simulink model "hf_point_mass_subsonic_airplane"  (R2024b)
settings: Solver=ode45  StartTime=0.0  StopTime=5*60  RelTol=1e-3  AbsTol=1e-6
values from neighbouring files (symbols this model uses):
  FPS2MPH = 3600/5280    (= 0.681818181818)    [luckep2.m]
  RAD2DEG = 180/pi    (= 57.2957795131)    [luckep2.m]
undefined symbols (not defined in the file or in its folder): gd, ic, params
libraries: simulink_extras x5, dspstat3 x1, simulink x1
(part 2 of 2)

== matlab function hf_point_mass_subsonic_airplane/Vehicle Dynamics/Heading Rate Equation/F_app2/rni/get r_ni ==
  data: bank input; rni output; fpa input; heading input; we input; latitude input; longitude input
function rni = getrni(bank,fpa,heading, we, latitude, longitude)
x = [bank, fpa, heading];
C = [cosd(fpa)*cosd(heading) cosd(fpa)*sind(heading) -sind(fpa)
    sind(bank)*sind(fpa)*cosd(heading) - cosd(bank)*sind(heading) sind(bank)*sind(fpa)*sind(heading) + cosd(bank)*cosd(heading) sind(bank)*cosd(fpa)
    cosd(bank)*sind(fpa)*cosd(heading) + sind(bank)*sind(heading) cosd(bank)*sind(fpa)*sind(heading) - sind(bank)*cosd(heading) cosd(bank)*cosd(fpa)];

mat = C*[(we + latitude)*cosd(longitude); -longitude;-(we + latitude)*sind(longitude)];
rni = mat(3);

== matlab function hf_point_mass_subsonic_airplane/Vehicle Dynamics/Heading Rate Equation/F_app3/fapp3_term3/MATLAB Function2 ==
  data: longitude input; latitude input; heading input; w_e input; fapp3 output; altitude input; RE input; bank input; flight_path input
function fapp3 = getFapp3(longitude, latitude, heading, w_e, altitude, RE, bank, flight_path)
fapp3 = -w_e.^2 * (RE + altitude) * cosd(latitude) * (sind(latitude) * (...
    (cosd(bank)*sind(flight_path)*cosd(heading) + sind(bank)*sind(heading)) + ...
    cosd(latitude)*cosd(bank)*cosd(flight_path)));

== matlab function hf_point_mass_subsonic_airplane/Vehicle Dynamics/Heading Rate Equation/F_app3/qei/get qei ==
  data: bank input; qei output; fpa input; heading input; we input; latitude input; longitude input
function qei = getqei(bank,fpa,heading, we, latitude, longitude)
x = [bank, fpa, heading];
C = [cosd(fpa)*cosd(heading) cosd(fpa)*sind(heading) -sind(fpa)
    sind(bank)*sind(fpa)*cosd(heading) - cosd(bank)*sind(heading) sind(bank)*sind(fpa)*sind(heading) + cosd(bank)*cosd(heading) sind(bank)*cosd(fpa)
    cosd(bank)*sind(fpa)*cosd(heading) + sind(bank)*sind(heading) cosd(bank)*sind(fpa)*sind(heading) - sind(bank)*cosd(heading) cosd(bank)*cosd(fpa)];

mat = C*[(we)*cosd(longitude); 0;-(we)*sind(longitude)];
qei = mat(2);

== matlab function hf_point_mass_subsonic_airplane/Vehicle Dynamics/Heading Rate Equation/F_app3/qni/get qni ==
  data: bank input; qni output; fpa input; heading input; we input; latitude input; longitude input
function qni = getqni(bank,fpa,heading, we, latitude, longitude)
x = [bank, fpa, heading];
C = [cosd(fpa)*cosd(heading) cosd(fpa)*sind(heading) -sind(fpa)
    sind(bank)*sind(fpa)*cosd(heading) - cosd(bank)*sind(heading) sind(bank)*sind(fpa)*sind(heading) + cosd(bank)*cosd(heading) sind(bank)*cosd(fpa)
    cosd(bank)*sind(fpa)*cosd(heading) + sind(bank)*sind(heading) cosd(bank)*sind(fpa)*sind(heading) - sind(bank)*cosd(heading) cosd(bank)*cosd(fpa)];

mat = C*[(we + latitude)*cosd(longitude); -longitude;-(we + latitude)*sind(longitude)];
qni = mat(2);

== matlab function hf_point_mass_subsonic_airplane/Vehicle Dynamics/Flight Path Rate Equation/MATLAB Function ==
  data: fapp2 input; fapp3 input; groundspeed input; flight_path_out output; mass input; lift input; bank input; gamma input; g input
function flight_path_out = getFlightPath(fapp2, fapp3, groundspeed, mass, lift,  bank, gamma, g)
flight_path_out = 1/groundspeed * (lift/mass*cosd(bank) - ...
    g * cosd(gamma) - (fapp2*sind(bank)+ fapp3*cosd(bank)));

== matlab function hf_point_mass_subsonic_airplane/Vehicle Dynamics/Heading Rate Equation/MATLAB Function ==
  data: fapp2 input; fapp3 input; flight_path input; heading_out output; groundspeed input; mass input; lift input; bank input
function heading_out = getHeading(fapp2, fapp3, flight_path, groundspeed, mass, lift,  bank)
heading_out = 1/(groundspeed*cosd(flight_path)) * (lift/mass*sind(bank));

== matlab function hf_point_mass_subsonic_airplane/Vehicle Dynamics/Inertial Position and Airspeed/MATLAB Function ==
  data: groundspeed input; hdot output; flight_path input
function hdot = calchdot(groundspeed, flight_path)
hdot = groundspeed * sind(flight_path);

== matlab function hf_point_mass_subsonic_airplane/Vehicle Dynamics/Inertial Position and Airspeed/MATLAB Function1 ==
  data: h input; groundspeed input; ldot output; flight_path input; heading input; RE input
function ldot = calc_ldot(h, groundspeed, flight_path, heading, RE)
ldot = groundspeed * cosd(flight_path)*cosd(heading)/(RE + h);

== matlab function hf_point_mass_subsonic_airplane/Vehicle Dynamics/Inertial Position and Airspeed/MATLAB Function2 ==
  data: h input; lambda_dot output; groundspeed input; flight_path input; heading input; longitude input; RE input
function lambda_dot = calcLambdaDot(h, groundspeed, flight_path, heading, longitude, RE)
lambda_dot = groundspeed * cosd(flight_path) * sind(heading)/...
    ((RE + h)*cosd(longitude));

== matlab function hf_point_mass_subsonic_airplane/Vehicle Dynamics/Inertial Position and Airspeed/MATLAB Function3 ==
  data: groundspeed input; aspeed output; fpa input; heading input; vwind input
function aspeed = getAirspeed(groundspeed, fpa, heading, vwind)
uvw = [groundspeed*cosd(fpa)*cosd(heading)
    groundspeed*cosd(fpa)*sind(heading)
    groundspeed*sind(fpa)];
vinf = uvw - [40 40 0]';
aspeed = vinf(1).^2 + vinf(2).^2 + vinf(3).^2;
